simulink model "P_controller"  (R2018a)
settings: Solver=VariableStepAuto  StartTime=0.0  StopTime=100  RelTol=1e-3
settings Model: Creator=mjb15180  LastModifiedBy=mjb15180

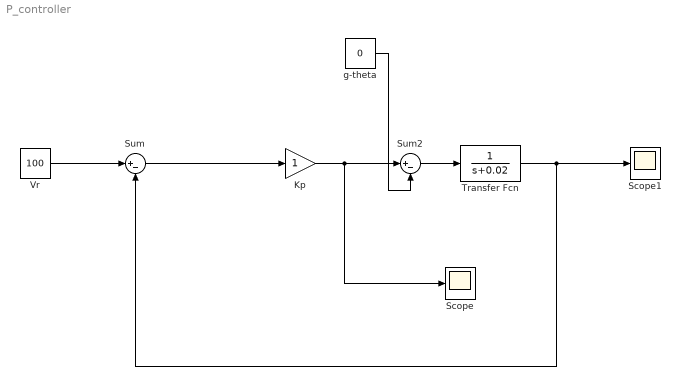
== system P_controller ==
  Kp : Gain
  Scope : Scope
  Scope1 : Scope
  Sum : Sum  Inputs=|+-
  Sum2 : Sum  Inputs=|+-
  Transfer Fcn : TransferFcn  Denominator=[1 0.02]
  Vr : Constant  Value=100
  g-theta : Constant  Value=0
  wires:
  Sum2/1 -> Transfer Fcn/1
  Transfer Fcn/1 -> Sum/2, Scope1/1
  Kp/1 -> Sum2/1, Scope/1
  g-theta/1 -> Sum2/2
  Sum/1 -> Kp/1
  Vr/1 -> Sum/1
